simulink model "yaw_controller"  (R2016b)
settings: Solver=VariableStepAuto  StartTime=0.0  StopTime=10.0  RelTol=1e-3
undefined symbols (not defined in the file): aa, b, b0, beta, beta1, d, delta, h, h0, r
settings Model: Creator=lvhuitao  LastModifiedBy=lvhuitao

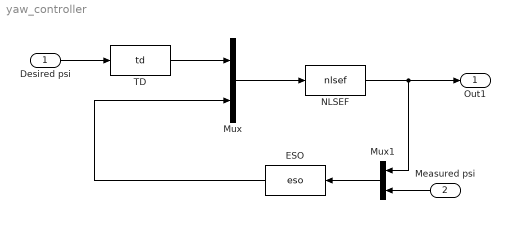
== system yaw_controller ==
  Desired psi : Inport
  Measured psi : Inport  Port=2
  ESO : S-Function  FunctionName=eso  Parameters=delta,beta,b0,h  SFunctionDeploymentMode=off  EnableBusSupport=off
  Mux : Mux  Inputs=2
  Mux1 : Mux  Inputs=2
  NLSEF : S-Function  FunctionName=nlsef  Parameters=aa,beta1,b,d  SFunctionDeploymentMode=off  EnableBusSupport=off
  TD : S-Function  FunctionName=td  Parameters=r,h0,h  SFunctionDeploymentMode=off  EnableBusSupport=off
  Out1 : Outport
  wires:
  Measured psi/1 -> Mux1/2
  Mux1/1 -> ESO/1
  ESO/1 -> Mux/2
  Desired psi/1 -> TD/1
  TD/1 -> Mux/1
  Mux/1 -> NLSEF/1
  NLSEF/1 -> Mux1/1, Out1/1
